simulink model "lab5_1_bad"  (R2015b)
settings: Solver=FixedStepDiscrete  StartTime=0.0  StopTime=inf  FixedStep=0.1  RelTol=1e-3
libraries: arduinolib x1
settings Model: ExtModeEnableFloating=off  ExtModeTrigDuration=2  ExtModeArchiveMode=auto  ExtModeArchiveFileName=data.mat  ExtModeArchiveDirName=/Users/kando/Google Drive/thesis/2017.03.14 Plant model parameterization/2. Data  ExtModeWriteAllDataToWs=on  Creator=kando  LastModifiedBy=kando
settings DataIOCC: LimitDataPoints=off  SaveOutput=off  SignalLogging=off  DSMLogging=off  VisualizeSimOutput=off  SaveTime=off
settings OptimizationCC: OptimizeModelRefInitCode=on  LifeSpan=Inf  MaxStackSize=64
settings HardwareCC: ProdBitPerInt=16  ProdBitPerPointer=16  ProdLargestAtomicFloat=None  ProdWordSize=8  ProdHWDeviceType=Atmel->AVR
settings RTWCC: SystemTargetFile=ert.tlc  TemplateMakefile=ert_default_tmf  Description=Embedded Coder  Toolchain=Arduino AVR v1.6.1  BuildConfiguration=Faster Runs
settings CodeAppCC: IgnoreCustomStorageClasses=off
settings ERTTargetCC: SupportContinuousTime=on  SupportVariableSizeSignals=on  ExtModeMexArgs=1 '/dev/cu.usbmodem621' 115200

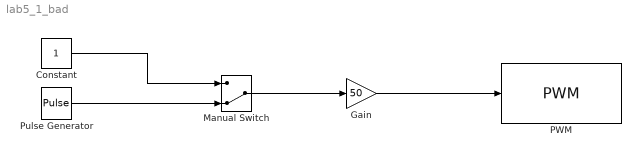
== system lab5_1_bad ==
  Constant : Constant
  Gain : Gain  Gain=50
  Manual Switch : ManualSwitch  CurrentSetting=0
  PWM : arduinolib/PWM  pinNumber=13  blockPlatform=arduino
  Pulse Generator : DiscretePulseGenerator  PulseType=Time based  PulseWidth=50
  wires:
  Pulse Generator/1 -> Manual Switch/2
  Constant/1 -> Manual Switch/1
  Manual Switch/1 -> Gain/1
  Gain/1 -> PWM/1
